simulink model "lookupnddirect_out_table_multi_test"  (Simulink 8.4)
settings: Solver=ode45  StartTime=0.0  StopTime=10.0  RelTol=1e-3
settings Model: Creator=arnaud  LastModifiedBy=arnaud
settings DataIOCC: SaveFormat=Structure

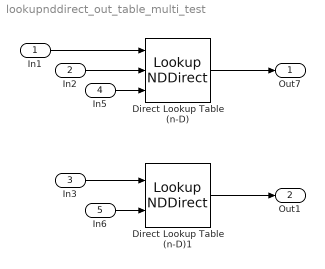
== system lookupnddirect_out_table_multi_test ==
  In1 : Inport  PortDimensions=2
  In2 : Inport  Port=2  PortDimensions=2
  In3 : Inport  Port=3  PortDimensions=2
  In5 : Inport  Port=4  PortDimensions=[2 3]
  In6 : Inport  Port=5  PortDimensions=4
  Direct Lookup Table (n-D) : LookupNDDirect  TableIsInput=on
  Direct Lookup Table (n-D)1 : LookupNDDirect  NumberOfTableDimensions=1  TableIsInput=on  Table=[4 5 6]
  Out7 : Outport
  Out1 : Outport  Port=2
  wires:
  In1/1 -> Direct Lookup Table (n-D)/1
  In2/1 -> Direct Lookup Table (n-D)/2
  Direct Lookup Table (n-D)/1 -> Out7/1
  In3/1 -> Direct Lookup Table (n-D)1/1
  Direct Lookup Table (n-D)1/1 -> Out1/1
  In5/1 -> Direct Lookup Table (n-D)/3
  In6/1 -> Direct Lookup Table (n-D)1/2
